simulink model "PIL_TopModel_dsPIC33CK_Curiosity"  (R2020b)
settings: Solver=FixedStepDiscrete  StartTime=0.0  StopTime=66  FixedStep=0.01  RelTol=1e-3
settings Model: ExtModeTrigDuration=1  Creator=M17129  LastModifiedBy=Lubin Kerhuel
settings DataIOCC: ReturnWorkspaceOutputs=off
settings OptimizationCC: DefaultParameterBehavior=Inlined  DefaultUnderspecifiedDataType=single  PassReuseOutputArgsAs=Individual arguments  EfficientTunableParamExpr=on
settings DebuggingCC: ParameterTunabilityLossMsg=error  ArithmeticOperatorsInVariantConditions=warning
settings HardwareCC: ProdBitPerInt=16  ProdBitPerPointer=16  ProdBitPerSizeT=16  ProdBitPerPtrDiffT=16  ProdLargestAtomicInteger=Integer  ProdLargestAtomicFloat=None  ProdWordSize=16  ProdHWDeviceType=Generic->Custom
settings ModelReferenceCC: ModelReferenceNumInstancesAllowed=Single  PropagateSignalLabelsOutOfModel=off
settings SFSimCC: SimUseLocalCustomCode=off  MATLABDynamicMemAlloc=off  CustomCodeUndefinedFunction=UseInterfaceOnly
settings RTWCC: Description=Microchip Embedded Target PIC24 dsPIC30 dsPIC33 (real-time)  SystemTargetFile=MCHP_dsPIC_stf.tlc  TemplateMakefile=MCHP_dsPIC.tmf  GenerateReport=on  RTWUseLocalCustomCode=off  IncludeHyperlinkInReport=on  LaunchReport=on  CodeExecutionProfiling=on  CodeProfilingSaveOptions=AllData  CodeProfilingInstrumentation=detailed  GenerateTraceInfo=on  GenerateTraceReport=on  GenerateTraceReportSl=on  GenerateTraceReportSf=on  GenerateTraceReportEml=on  GenerateWebview=on  GenerateCodeMetricsReport=on  GenerateCodeReplacementReport=on
settings CodeAppCC: ForceParamTrailComments=on  IgnoreCustomStorageClasses=off  MaxIdLength=255  OperatorAnnotations=on  SimulinkDataObjDesc=on  SFDataObjDesc=on  InsertBlockDesc=on
settings STFCustomTargetCC: TargetLibSuffix=_lib.a  CodeReplacementLibrary=Microchip Code Replacement Library for dsPIC  MultiwordLength=256  ConcurrentExecutionCompliant=off  IncludeMdlTerminateFcn=off  CombineOutputUpdateFcns=on  SuppressErrorStatus=on  ERTCustomFileBanners=on  SupportContinuousTime=off  MATLABClassNameForMDSCustomization=Simulink.SoftwareTarget.ERTCustomization  CPPClassGenCompliant=off  GRTInterface=off  SystemTargetFile=MCHP_dsPIC_stf.tlc
settings ERTTargetCC: TargetLibSuffix=_lib.a  CodeReplacementLibrary=Microchip Code Replacement Library for dsPIC  ParMdlRefBuildCompliant=off  CompOptLevelCompliant=off  ConcurrentExecutionCompliant=off  IncludeMdlTerminateFcn=off  SuppressErrorStatus=on  SupportNonInlinedSFcns=on  RemoveResetFunc=off  ModelStepFunctionPrototypeControlCompliant=off  CPPClassGenCompliant=off  UseToolchainInfoCompliant=off  ExtModeTransport=1  ExtModeStaticAllocSize=500  ExtModeMexFile=ext_xcp  ExtModeMexArgs=0 0 115200  ExtModeIntrfLevel=Level2 - Open  InlinedParameterPlacement=NonHierarchical  ERTSrcFileBannerTemplate=MCHP_dsPIC_code_template.cgt  ERTHdrFileBannerTemplate=MCHP_dsPIC_code_template.cgt  ERTDataSrcFileTemplate=MCHP_dsPIC_code_template.cgt  ERTDataHdrFileTemplate=MCHP_dsPIC_code_template.cgt  ERTCustomFileTemplate=MCHP_main.tlc

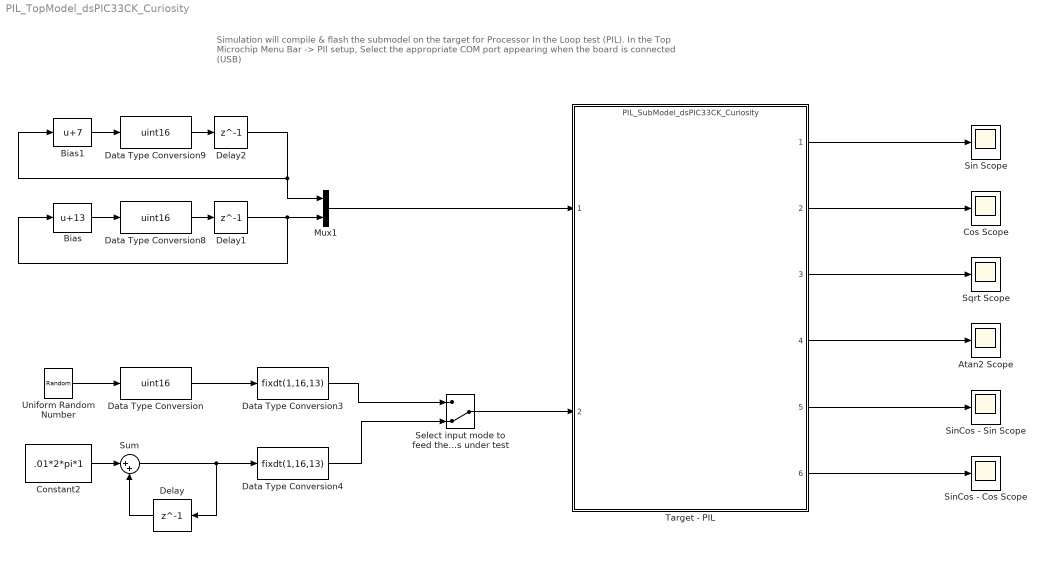
== system PIL_TopModel_dsPIC33CK_Curiosity ==
  note: Simulation will compile & flash the submodel on the target for Processor In the Loop test (PIL).
      | In the Top Microchip Menu Bar -> PIl setup, Select the appropriate COM port appearing when the board is connected (USB)
  Atan2 Scope : Scope
  Bias : Bias  Bias=13
  Bias1 : Bias  Bias=7
  Constant2 : Constant  Value=.01*2*pi*1  OutDataTypeStr=fixdt(1,16,2*pi/65536,0)  SampleTime=.01
  Cos Scope : Scope
  Data Type Conversion : DataTypeConversion  OutDataTypeStr=uint16  ConvertRealWorld=Stored Integer (SI)
  Data Type Conversion3 : DataTypeConversion  OutDataTypeStr=fixdt(1,16,13)  ConvertRealWorld=Stored Integer (SI)
  Data Type Conversion4 : DataTypeConversion  OutDataTypeStr=fixdt(1,16,13)
  Data Type Conversion8 : DataTypeConversion  OutDataTypeStr=uint16  ConvertRealWorld=Stored Integer (SI)
  Data Type Conversion9 : DataTypeConversion  OutDataTypeStr=uint16  ConvertRealWorld=Stored Integer (SI)
  Delay : Delay  DelayLength=1  InitialCondition=0
  Delay1 : Delay  DelayLength=1  InitialCondition=0
  Delay2 : Delay  DelayLength=1  InitialCondition=0
  Mux1 : Mux  Inputs=2
  Select input mode to feed the functions under test : ManualSwitch  CurrentSetting=0
  Sin Scope : Scope
  "SinCos - Cos Scope " : Scope
  SinCos - Sin Scope : Scope
  Sqrt Scope : Scope
  Sum : Sum  Inputs=|++  OutDataTypeStr=Inherit: Same as first input
  Target - PIL : ModelReference  ModelNameDialog=PIL_SubModel_dsPIC33CK_Curiosity.slx  SimulationMode=Processor-in-the-loop (PIL)  ModelReferenceVersion=7.11
  Uniform Random Number : UniformRandomNumber  Minimum=0  Maximum=2^16-1  SampleTime=.01
  wires:
  Target - PIL/1 -> Sin Scope/1
  Target - PIL/2 -> Cos Scope/1
  Target - PIL/3 -> Sqrt Scope/1
  Target - PIL/4 -> Atan2 Scope/1
  Target - PIL/5 -> SinCos - Sin Scope/1
  Target - PIL/6 -> "SinCos - Cos Scope "/1
  Data Type Conversion/1 -> Data Type Conversion3/1
  Constant2/1 -> Sum/1
  Data Type Conversion4/1 -> Select input mode to feed the functions under test/2
  Data Type Conversion3/1 -> Select input mode to feed the functions under test/1
  Uniform Random Number/1 -> Data Type Conversion/1
  Delay/1 -> Sum/2
  Sum/1 -> Data Type Conversion4/1, Delay/1
  Select input mode to feed the functions under test/1 -> Target - PIL/2
  Mux1/1 -> Target - PIL/1
  Delay2/1 -> Mux1/1, Bias1/1
  Delay1/1 -> Bias/1, Mux1/2
  Data Type Conversion8/1 -> Delay1/1
  Bias/1 -> Data Type Conversion8/1
  Data Type Conversion9/1 -> Delay2/1
  Bias1/1 -> Data Type Conversion9/1
